simulink model "exampleModel_bus_axi_w_4ptavg"  (R2017b)
settings: Solver=VariableStepAuto  StartTime=0.0  StopTime=10e-5  RelTol=1e-3
PreLoadFcn:
  | setup
values from neighbouring files (symbols this model uses):
  axiClk = 156.25e6    (= 156250000)    [setup.m]    (also in setup_exampleModel_bus_axi_simulink.m; setup_exampleModel_bus_axi_simulink_lcls2.m; setup_lcls2_pcav.m; sysgen_signal.m)
  cav1p1_addr = 204    [setup_exampleModel_bus_axi_simulink.m]    (also in setup_exampleModel_bus_axi_simulink_lcls2.m; setup_lcls2_pcav.m; sysgen_signal.m)
  cav1p2_addr = cav1p1_addr * 2    (= 408)    [setup_exampleModel_bus_axi_simulink.m]    (also in setup_exampleModel_bus_axi_simulink_lcls2.m; setup_lcls2_pcav.m; sysgen_signal.m)
  cav2p1_addr = cav1p1_addr * 3    (= 612)    [setup_exampleModel_bus_axi_simulink.m]    (also in setup_exampleModel_bus_axi_simulink_lcls2.m; setup_lcls2_pcav.m; sysgen_signal.m)
  cav2p2_addr = cav1p1_addr * 4    (= 816)    [setup_exampleModel_bus_axi_simulink.m]    (also in setup_exampleModel_bus_axi_simulink_lcls2.m; setup_lcls2_pcav.m; sysgen_signal.m)
  Fadc = Fs/interleavedChannels    (= 29750000)    [setup.m]    (also in setup_exampleModel_bus_axi_simulink.m = 357000000; setup_exampleModel_bus_axi_simulink_lcls2.m = 351000000; setup_lcls2_pcav.m = 357000000; sysgen_signal.m = 357000000)
  fir_lpf = fir1(15, w_lpf)    [setup_exampleModel_bus_axi_simulink.m]    (also in setup_exampleModel_bus_axi_simulink_lcls2.m; setup_lcls2_pcav.m)
  Fproc = 204e6    (= 204000000)    [setup_exampleModel_bus_axi_simulink.m]    (also in setup_exampleModel_bus_axi_simulink_lcls2.m = 200571400; setup_lcls2_pcav.m; sysgen_signal.m)
  Fsig = Fproc/12    (= 17000000)    [setup_exampleModel_bus_axi_simulink.m]    (also in setup_exampleModel_bus_axi_simulink_lcls2.m = 16714283.3333; setup_lcls2_pcav.m)
  Tadc = 1/fadc    (= 2.80112044818e-09)    [cavity_signal.m]    (also in setup_exampleModel_bus_axi_simulink.m; setup_exampleModel_bus_axi_simulink_lcls2.m = 2.849002849e-09; setup_lcls2_pcav.m; setup_pcav_simulink.m)
undefined symbols (not defined in the file or in its folder): AXI4, Lite
libraries: xbsIndex_r4 x2870, llrf_lib x10, simulink x3
(part 5 of 15)

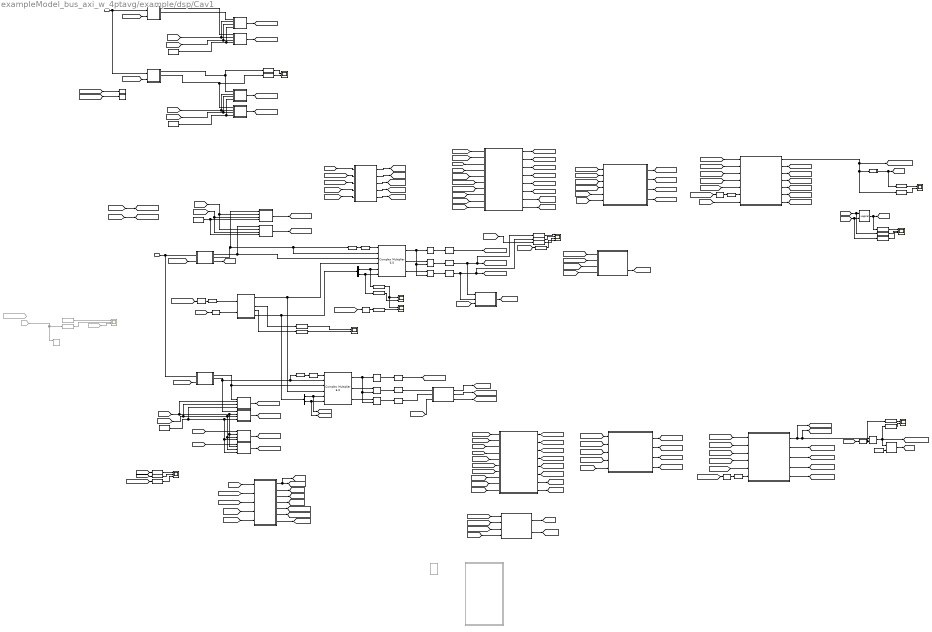
== system exampleModel_bus_axi_w_4ptavg/example/dsp/Cav1 ==
  PA_stream : Inport
  IQ_stream : Inport  Port=2
  AddSub : xbsIndex_r4/AddSub  Commented=on  mode=Addition  use_carryin=off  use_carryout=off  en=off  latency=1  precision=User Defined  arith_type=Unsigned  n_bits=32  bin_pt=32  quantization=Truncate  overflow=Saturate  use_behavioral_HDL=off  hw_selection=Fabric  pipelined=off  dbl_ovrd=off  block_type=addsub
  Bus Selector : BusSelector  OutputSignals=NCO_sin,NCO_cos
  Bus Selector1 : BusSelector  OutputSignals=NCO_sin,NCO_cos
  Clock Enable Probe : xbsIndex_r4/Clock Enable Probe  inherit_constraints=on  block_type=ceprobe
      settings: infoedit="Clock enable extractor.  Produces a Boolean output that mirrors the hardware clock enable associated with the input sample rate.<br><br>Hardware notes: in hardware this block costs nothing."
  Clock Enable Probe1 : xbsIndex_r4/Clock Enable Probe  inherit_constraints=on  block_type=ceprobe
      settings: infoedit="Clock enable extractor.  Produces a Boolean output that mirrors the hardware clock enable associated with the input sample rate.<br><br>Hardware notes: in hardware this block costs nothing."
  "Complex Multiplier 6.0 " : xbsIndex_r4/Complex Multiplier 6.0   hasatlast=off  hasatuser=off  atuserwidth=1  hasbtlast=off  hasbtuser=off  btuserwidth=1  multtype=Use_Mults  optimizegoal=Resources  flowcontrol=NonBlocking  outputwidth=33  roundmode=Truncate  hasctrltlast=off  hasctrltuser=off  ctrltuserwidth=1  outtlastbehv=Null  latencyconfig=Automatic  minimumlatency=15  aclken=off  aresetn=off  trim_axipin_name=on  simulation_type=hybrid_sim  simulation_model=sysgen:cmpy_v6_0  data_path_portlist={ 's_axis_a_tdata_real', 's_axis_a_tdata_imag', 's_axis_b_tdata_real', 's_axis_b_tdata_imag', 's_axis_ctrl_tdata_rounding_bit', 'm_axis_dout_tdata_real', 'm_axis_dout_tdata_imag' }  aportwidth=63  bportwidth=63  ip_name=Complex Multiplier  ip_version=6.0  dsptool_ready=true  ipcore_usecache=true  ipcore_useipmodelcache=true  ipcore_verbose=false  ipcore_latency_parameter='minimumlatency'  wrapper_available=true  port_translation_map={ 'aclken' => 'en', 'aresetn' => 'rst'}  block_type=cmpy_v6_0
  Complex Multiplier 6.0 1 : xbsIndex_r4/Complex Multiplier 6.0   hasatlast=off  hasatuser=off  atuserwidth=1  hasbtlast=off  hasbtuser=off  btuserwidth=1  multtype=Use_Mults  optimizegoal=Resources  flowcontrol=NonBlocking  outputwidth=21  roundmode=Truncate  hasctrltlast=off  hasctrltuser=off  ctrltuserwidth=1  outtlastbehv=Null  latencyconfig=Automatic  minimumlatency=37  aclken=off  aresetn=off  trim_axipin_name=on  simulation_type=hybrid_sim  simulation_model=sysgen:cmpy_v6_0  data_path_portlist={ 's_axis_a_tdata_real', 's_axis_a_tdata_imag', 's_axis_b_tdata_real', 's_axis_b_tdata_imag', 's_axis_ctrl_tdata_rounding_bit', 'm_axis_dout_tdata_real', 'm_axis_dout_tdata_imag' }  aportwidth=63  bportwidth=63  ip_name=Complex Multiplier  ip_version=6.0  dsptool_ready=true  ipcore_usecache=true  ipcore_useipmodelcache=true  ipcore_verbose=false  ipcore_latency_parameter='minimumlatency'  wrapper_available=true  port_translation_map={ 'aclken' => 'en', 'aresetn' => 'rst'}  block_type=cmpy_v6_0
  Constant : xbsIndex_r4/Constant  const=0  gui_display_data_type=Fixed-point  arith_type=Signed (2's comp)  n_bits=1  bin_pt=0  preci_type=Single  exp_width=8  frac_width=24  explicit_period=off  period=1  equ=P=C  opselect=C  inp2=PCIN>>17  opr=+  inp1=P  carry=CIN  dbl_ovrd=off  block_type=constant
  Constant{1..4} (4 alike) : xbsIndex_r4/Constant  const=29  gui_display_data_type=Fixed-point  arith_type=Unsigned  n_bits=16  bin_pt=0  preci_type=Single  exp_width=8  frac_width=24  explicit_period=off  period=1  equ=P=C  opselect=C  inp2=PCIN>>17  opr=+  inp1=P  carry=CIN  dbl_ovrd=off  block_type=constant
  Convert{,1,5..6} (4 alike) : xbsIndex_r4/Convert  gui_display_data_type=Fixed-point  arith_type="Signed  (2's comp)"  n_bits=18  bin_pt=16  float_type=Single  exp_bits=8  fraction_bits=24  quantization=Truncate  overflow=Wrap  en=off  latency=1  pipeline=off  dbl_ovrd=off  block_type=convert
  Convert10 : xbsIndex_r4/Convert  gui_display_data_type=Boolean  arith_type=Boolean  n_bits=16  bin_pt=14  float_type=Single  exp_bits=8  fraction_bits=24  quantization=Truncate  overflow=Wrap  en=off  latency=1  pipeline=off  dbl_ovrd=off  block_type=convert
  Convert2 : xbsIndex_r4/Convert  gui_display_data_type=Boolean  arith_type=Boolean  n_bits=18  bin_pt=16  float_type=Single  exp_bits=8  fraction_bits=24  quantization=Truncate  overflow=Wrap  en=off  latency=1  pipeline=off  dbl_ovrd=off  block_type=convert
  Convert9 : xbsIndex_r4/Convert  gui_display_data_type=Boolean  arith_type=Boolean  n_bits=18  bin_pt=16  float_type=Single  exp_bits=8  fraction_bits=24  quantization=Truncate  overflow=Wrap  en=off  latency=1  pipeline=off  dbl_ovrd=off  block_type=convert
  DDC NCO1 : Subsystem
  Down Sample{1..3,6..7} (5 alike) : xbsIndex_r4/Down Sample  sample_ratio=12  sample_phase="Last Value of Frame  (most efficient)"  en=off  rst=off  latency=1  dbl_ovrd=off  block_type=dsamp
  From89 : From  Commented=on  GotoTag=cav1_p2_dc_freq  TagVisibility=global
  From90 : From  Commented=on  GotoTag=sim_f_err  TagVisibility=global
  From91 : From  Commented=on  GotoTag=testa  TagVisibility=global
  Gateway Out{1..6,8..10,25,39..40} (12 alike) : xbsIndex_r4/Gateway Out  inherit_from_input=off  hdl_port=on  rows=1  columns=1  UseAsDAC=off  DACChannel='1'  interface=None  automatic_assignment=on  address_offset=hex2dec('00')  intf_name=''  intf_description=''  timing_constraint=None  locs_specified=off  LOCs={}  io_standard={}  block_type=gatewayout
  Gateway Out{26..28,30..33} (7 alike) : xbsIndex_r4/Gateway Out  inherit_from_input=off  hdl_port=off  rows=1  columns=1  UseAsDAC=off  DACChannel='1'  interface=None  automatic_assignment=on  address_offset=hex2dec('00')  intf_name=''  intf_description=''  timing_constraint=None  locs_specified=off  LOCs={}  io_standard={}  block_type=gatewayout
  Gateway Out36 : xbsIndex_r4/Gateway Out  Commented=on  inherit_from_input=off  hdl_port=on  rows=1  columns=1  UseAsDAC=off  DACChannel='1'  interface=None  automatic_assignment=on  address_offset=hex2dec('00')  intf_name=''  intf_description=''  timing_constraint=None  locs_specified=off  LOCs={}  io_standard={}  block_type=gatewayout
  Gateway Out37 : xbsIndex_r4/Gateway Out  Commented=on  inherit_from_input=off  hdl_port=on  rows=1  columns=1  UseAsDAC=off  DACChannel='1'  interface=None  automatic_assignment=on  address_offset=hex2dec('00')  intf_name=''  intf_description=''  timing_constraint=None  locs_specified=off  LOCs={}  io_standard={}  block_type=gatewayout
  IQ_integration : Subsystem
  IQ_integration1 : Subsystem
  Logical : xbsIndex_r4/Logical  logical_function=AND  inputs=2  en=off  latency=1  precision=Full  arith_type=Unsigned  n_bits=16  bin_pt=0  align_bp=on  dbl_ovrd=off  block_type=logical
  Masking_n_delay : Subsystem
  NCO_cos : xbsIndex_r4/Gateway Out  inherit_from_input=off  hdl_port=off  rows=1  columns=1  UseAsDAC=off  DACChannel='1'  interface=None  automatic_assignment=on  address_offset=hex2dec('00')  intf_name=''  intf_description=''  timing_constraint=None  locs_specified=off  LOCs={}  io_standard={}  block_type=gatewayout
  NCO_sin : xbsIndex_r4/Gateway Out  inherit_from_input=off  hdl_port=off  rows=1  columns=1  UseAsDAC=off  DACChannel='1'  interface=None  automatic_assignment=on  address_offset=hex2dec('00')  intf_name=''  intf_description=''  timing_constraint=None  locs_specified=off  LOCs={}  io_standard={}  block_type=gatewayout
  PA_conversion2 : Subsystem
  PA_select : Subsystem
  PA_select1 : Subsystem
  Register : xbsIndex_r4/Register  init=0  rst=on  en=off  dbl_ovrd=off  block_type=register
  Register{1..2,32..33} (4 alike) : xbsIndex_r4/Register  init=0  rst=off  en=on  dbl_ovrd=off  block_type=register
  Register{3..10,31} (9 alike) : xbsIndex_r4/Register  init=0  rst=off  en=off  dbl_ovrd=off  block_type=register
  Relational : xbsIndex_r4/Relational  mode=a!=b  op_type=Bool  en=off  latency=1  dbl_ovrd=off  block_type=relational
  Scope1 : Scope  NumInputPorts=4
  Scope{2..3,11..14} (6 alike) : Scope  NumInputPorts=2
  Scope15 : Scope  NumInputPorts=3
  Scope17 : Scope  Commented=on  NumInputPorts=3
  Scope18 : Scope  NumInputPorts=3
  Subsystem : Subsystem  Commented=on
  Subsystem1 : Subsystem
  Subsystem10 : Subsystem
  Subsystem11 : Subsystem
  Subsystem12 : Subsystem
  Subsystem13 : Subsystem
  Subsystem2 : Subsystem
  Subsystem3 : Subsystem
  Subsystem4 : Subsystem
  Subsystem5 : Subsystem
  Subsystem6 : Subsystem
  Subsystem7 : Subsystem
  Subsystem8 : Subsystem
  Subsystem9 : Subsystem
  c1p1_Masking_window : Subsystem
  c1p1_PA_conversion : Subsystem
  c1p1_freq_err_module : Subsystem
  "c1p1_window_wf1 " : Subsystem
  c1p2_freq_err_module : Subsystem
  c1p2_window_wf : Subsystem
  c1p2_window_wf1 : Subsystem  Commented=on
  c1p2_windowing_func1 : Subsystem
  c1p2_windowing_func2 : Subsystem
  tag scope: Cav1_NCO_fb=global, c1_p1_delay_amt=global, c1_p1_delay_latch=global, c1_p2_delay_amt=global, c1_p2_delay_latch=global, c1_ready=global, c1_stream_valid=global, c1p1_delay_match=global, c1p1_freq_err=global, c1p1_integral_logic=global, c1p1_pt_cntr=global, c1p1_pt_window=global, c1p1_ready=global, c1p1_window_func=global, c1p2_delay_match=global, c1p2_freq_err=global, c1p2_integral_logic=global, c1p2_pt_cntr=global, c1p2_pt_window=global, c1p2_ready=global, c1p2_window_func=global, cav1_NCO_cos=global, cav1_NCO_sin=global, cav1_p1_amp_out=global, cav1_p1_comparison_i=global, cav1_p1_comparison_phase=global, cav1_p1_comparison_q=global, cav1_p1_dc_freq=global, cav1_p1_dc_img=global, cav1_p1_dc_real=global, cav1_p1_dc_tvalid=global, cav1_p1_delayed_dc_img=global, cav1_p1_delayed_dc_real=global, cav1_p1_if_amp=global, cav1_p1_if_i=global, cav1_p1_if_phase=global, cav1_p1_if_q=global, cav1_p1_integrated_i=global, cav1_p1_integrated_q=global, cav1_p1_integrated_ref_i=global, cav1_p1_integrated_ref_q=global, cav1_p1_phase_out=global, cav1_p1_ref_amp_out=global, cav1_p1_ref_phase_out=global, cav1_p1_windowed_img=global, cav1_p1_windowed_real=global, cav1_p1_windowed_ref_i=global, cav1_p1_windowed_ref_q=global, cav1_p2_amp_out=global, cav1_p2_comparison_i=global, cav1_p2_comparison_phase=global, cav1_p2_comparison_q=global, cav1_p2_dc_freq=global, cav1_p2_dc_img=global, cav1_p2_dc_real=global, cav1_p2_dc_tvalid=global, cav1_p2_delayed_dc_img=global, cav1_p2_delayed_dc_real=global, cav1_p2_if_amp=global, cav1_p2_if_i=global, cav1_p2_if_phase=global, cav1_p2_if_q=global, cav1_p2_integrated_i=global, cav1_p2_integrated_q=global, cav1_p2_integrated_ref_i=global, cav1_p2_integrated_ref_q=global, cav1_p2_phase_out=global, cav1_p2_ref_amp_out=global, cav1_p2_ref_phase_out=global, cav1_p2_windowed_img=global, cav1_p2_windowed_real=global, cav1_p2_windowed_ref_i=global, cav1_p2_windowed_ref_q=global, cav1_sync=global, dsp_cav1_reset=global, flo_c1p1_window=global, flo_c1p2_window=global, ref_i_reg=global, ref_q_reg=global, reset=global
  wires:
  PA_select/1(Amp) -> Subsystem13/1(d)
  "Complex Multiplier 6.0 "/2 -> Register1/1
  Bus Selector/2 -> NCO_cos/1, "Complex Multiplier 6.0 "/6  "<NCO_cos>"
  "Complex Multiplier 6.0 "/3 -> Register2/1
  [cav1_nco_phase_adj] -> Register8/1
  [cav1_sync] -> Register7/1
  Bus Selector/1 -> NCO_sin/1, "Complex Multiplier 6.0 "/5  "<NCO_sin>"
  DDC NCO1/5(NCO_out) -> Bus Selector1/1, Bus Selector/1
  PA_select/2(Phase) -> Subsystem12/1(d)  "phase"
  Subsystem3/2(ddcQ) -> Subsystem6/1(d), "Complex Multiplier 6.0 "/2, Clock Enable Probe/1  "ddcQ"
  Subsystem3/1(ddcI) -> Subsystem7/1(d), "Complex Multiplier 6.0 "/3  "ddcI"
  NCO_cos/1 -> Scope11/2
  NCO_sin/1 -> Scope12/1, Scope11/1
  Clock Enable Probe/1 -> Down Sample2/1
  IQ_stream/1 -> Subsystem1/1(IQ_stream_in), Subsystem3/1(IQ_stream_in)
  [cav1_p1_chan_sel] -> PA_select/2(PA_chan_sel)
  [cav1_p1_chan_sel] -> Subsystem3/2(IQ_chan_sel)
  [cav1_nco_phase_adj] -> Register9/1
  [cav1_p2_chan_sel] -> PA_select1/2(PA_chan_sel)
  PA_select1/2(Phase) -> Gateway Out9/1, Subsystem11/1(d)  "phase"
  PA_select1/1(Amp) -> Gateway Out8/1, Subsystem10/1(d)
  PA_stream/1 -> PA_select1/1(PA_bus), PA_select/1(PA_bus)
  [cav1_p2_chan_sel] -> Subsystem1/2(IQ_chan_sel)
  Complex Multiplier 6.0 1/2 -> Register32/1
  Register31/1 -> Convert2/1
  Complex Multiplier 6.0 1/1 -> Register33/2, Register32/2, Register31/1
  Bus Selector1/2 -> [cav1_NCO_cos], Complex Multiplier 6.0 1/6  "<NCO_cos>"
  Bus Selector1/1 -> [cav1_NCO_sin], Complex Multiplier 6.0 1/5  "<NCO_sin>"
  Complex Multiplier 6.0 1/3 -> Register33/1
  [cav1_p1_window_start] -> Register3/1
  [cav1_p1_window_stop] -> Register4/1
  [c1p1_freq_err] -> [cav1_p1_dc_freq]
  [c1p2_freq_err] -> [cav1_p2_dc_freq]
  Convert/1 -> c1p2_windowing_func2/1(imag)
  Convert1/1 -> c1p2_windowing_func2/2(real)
  Convert2/1 -> [cav1_p2_dc_tvalid]
  Gateway Out4/1 -> Scope12/2
  Register8/1 -> Down Sample6/1
  Register9/1 -> Gateway Out4/1
  Gateway Out40/1 -> Scope18/2
  Gateway Out39/1 -> Scope18/1
  [rf_ref_amp] -> Gateway Out39/1
  [rf_ref_phase] -> Gateway Out40/1
  Register33/1 -> Convert1/1
  [c1p2_pt_window] -> IQ_integration/5(window_profile)
  [cav1_p2_windowed_ref_q] -> IQ_integration/4(ref_windowed_q)
  [cav1_p2_windowed_ref_i] -> IQ_integration/3(ref_windowed_i)
  [cav1_p2_windowed_real] -> IQ_integration/2(cav_windowed_real)
  [cav1_p2_windowed_img] -> IQ_integration/1(cav_windowed_imag)
  [cav1_sync] -> Masking_n_delay/1(phi_reset_trig)
  [cav1_p2_window_start] -> Masking_n_delay/2(start_pt)
  [cav1_p2_window_stop] -> Masking_n_delay/3(stop_pt)
  Masking_n_delay/1(trig_reset) -> [reset], [dsp_cav1_reset]
  Masking_n_delay/2(counter) -> [c1p2_pt_cntr]
  Masking_n_delay/3(eval_window) -> [c1p2_pt_window]
  Masking_n_delay/4(integral_trig) -> [c1p2_integral_logic]
  IQ_integration/4(ref_int_q) -> [cav1_p2_integrated_ref_q]
  IQ_integration/3(ref_int_i) -> [cav1_p2_integrated_ref_i]
  IQ_integration/2(cav_int_i) -> [cav1_p2_integrated_i]
  IQ_integration/1(cav_int_q) -> [cav1_p2_integrated_q]
  DDC NCO1/3(Sine) -> Gateway Out3/1
  DDC NCO1/4(Cosine) -> Gateway Out5/1
  Gateway Out3/1 -> Scope2/1
  Gateway Out5/1 -> Scope2/2
  Down Sample2/1 -> "Complex Multiplier 6.0 "/1
  Clock Enable Probe1/1 -> Down Sample1/1
  Down Sample1/1 -> Complex Multiplier 6.0 1/1
  Register7/1 -> DDC NCO1/2(Phase_reset)
  Convert5/1 -> c1p2_windowing_func1/1(imag), Gateway Out1/1, [cav1_p1_dc_img]
  Convert6/1 -> c1p2_windowing_func1/2(real), Gateway Out10/1, [cav1_p1_dc_real]
  [c1p1_pt_window] -> IQ_integration1/5(window_profile)
  IQ_integration1/2(cav_int_i) -> [cav1_p1_integrated_i]
  [cav1_p1_integrated_i] -> c1p1_PA_conversion/2(cav_int_i)
  [cav1_p1_windowed_ref_q] -> IQ_integration1/4(ref_windowed_q)
  Down Sample7/1 -> c1p1_PA_conversion/6(cal_coefficient)
  [cav1_p1_integrated_q] -> c1p1_PA_conversion/1(cav_int_q)
  IQ_integration1/3(ref_int_i) -> [cav1_p1_integrated_ref_i]
  [cav1_p1_integrated_ref_i] -> c1p1_PA_conversion/4(ref_int_i)
  Register6/1 -> Down Sample7/1
  [c1p1_integral_logic] -> c1p1_PA_conversion/5(integration_trig)
  [cav1_p1_windowed_img] -> IQ_integration1/1(cav_windowed_imag)
  [cav1_p1_cal_coef] -> Register6/1
  IQ_integration1/4(ref_int_q) -> [cav1_p1_integrated_ref_q]
  [cav1_p1_integrated_ref_q] -> c1p1_PA_conversion/3(ref_int_q)
  [cav1_p1_windowed_real] -> IQ_integration1/2(cav_windowed_real)
  [cav1_p1_windowed_ref_i] -> IQ_integration1/3(ref_windowed_i)
  IQ_integration1/1(cav_int_q) -> [cav1_p1_integrated_q]
  c1p1_Masking_window/2(eval_window) -> [c1p1_pt_window]
  [cav1_p1_window_start] -> c1p1_Masking_window/2(start_pt)
  [cav1_p1_window_stop] -> c1p1_Masking_window/3(stop_pt)
  [cav1_sync] -> c1p1_Masking_window/1(phi_reset_trig)
  c1p1_Masking_window/1(counter) -> [c1p1_pt_cntr]
  c1p1_Masking_window/3(integral_trig) -> [c1p1_integral_logic]
  Register1/1 -> Convert5/1
  Register2/1 -> Convert6/1
  "Complex Multiplier 6.0 "/1 -> Register10/1, Register2/2, Register1/2
  Register10/1 -> Convert9/1
  Convert9/1 -> [cav1_p1_dc_tvalid]
  c1p1_Masking_window/4(flo_window) -> [flo_c1p1_window]
  c1p1_PA_conversion/2(ref_phi_out) -> [cav1_p1_ref_phase_out]
  c1p1_PA_conversion/3(ref_amp_out) -> [cav1_p1_ref_amp_out]
  c1p1_PA_conversion/4(cav_phi_out) -> [cav1_p1_phase_out]
  c1p1_PA_conversion/5(cav_amp_out) -> [cav1_p1_amp_out]
  Masking_n_delay/5(flo_window) -> [flo_c1p2_window]
  [cav1_p2_dc_real] -> c1p2_window_wf/2(cav_real)
  [cav1_p2_dc_img] -> c1p2_window_wf/1(cav_img)
  [rf_ref_q] -> c1p2_window_wf/3(ref_img)
  [rf_ref_i] -> c1p2_window_wf/4(ref_real)
  [c1p2_window_func] -> c1p2_window_wf/5(window_profile)
  [cav1_p2_delayed_dc_real] -> c1p2_window_wf/7(cav_delayed_real)
  [cav1_p2_delayed_dc_img] -> c1p2_window_wf/6(cav_delayed_imag)
  [c1p2_pt_cntr] -> c1p2_window_wf/10(pt_cntr)
  [c1p2_pt_window] -> c1p2_window_wf/8(pt_window)
  [c1p2_delay_match] -> c1p2_window_wf/9(delay_match_amt)
  c1p2_window_wf/7(delay_amt) -> [c1_p2_delay_amt]
  c1p2_window_wf/1(cav_windowed_imag) -> [cav1_p2_windowed_img]
  c1p2_window_wf/2(cav_windowed_real) -> [cav1_p2_windowed_real]
  c1p2_window_wf/3(ref_windowed_imag) -> [cav1_p2_windowed_ref_q]
  c1p2_window_wf/4(ref_windowed_real) -> [cav1_p2_windowed_ref_i]
  c1p2_window_wf/5(delayed_cav_dc_img) -> [cav1_p2_delayed_dc_img]
  c1p2_window_wf/6(delayed_cav_dc_real) -> [cav1_p2_delayed_dc_real]
  [cav1_p2_integrated_ref_q] -> PA_conversion2/3(ref_int_q)
  [cav1_p2_integrated_i] -> PA_conversion2/2(cav_int_i)
  [cav1_p2_integrated_q] -> PA_conversion2/1(cav_int_q)
  [cav1_p2_integrated_ref_i] -> PA_conversion2/4(ref_int_i)
  Register5/1 -> Down Sample3/1
  [cav1_p2_cal_coef] -> Register5/1
  [c1p2_integral_logic] -> PA_conversion2/5(integration_trig)
  Down Sample3/1 -> PA_conversion2/6(cal_coefficient)
  PA_conversion2/1(phi_diff) -> [cav1_p2_comparison_q], Register/1, [cav1_p2_comparison_i]
  PA_conversion2/2(ref_phi_out) -> [cav1_p2_ref_phase_out]
  PA_conversion2/3(ref_amp_out) -> [cav1_p2_ref_amp_out]
  PA_conversion2/4(cav_phi_out) -> [cav1_p2_phase_out]
  PA_conversion2/5(cav_amp_out) -> [cav1_p2_amp_out]
  c1p2_windowing_func1/1(Window_profile) -> [c1p1_window_func]
  DDC NCO1/1(tvalid) -> "Complex Multiplier 6.0 "/4, Complex Multiplier 6.0 1/4
  Subsystem3/3(sync) -> [cav1_sync]  "sync"
  [cav1_nco_phase_reset] -> Gateway Out25/1
  Gateway Out25/1 -> Scope18/3
  [cav1_sync] -> Convert10/1
  Convert10/1 -> Gateway Out26/1, Register/2
  Gateway Out26/1 -> Scope13/1
  Gateway Out27/1 -> Scope13/2
  Register/1 -> [cav1_p2_comparison_phase], Relational/1, Gateway Out27/1
  Constant/1 -> Relational/2
  Relational/1 -> [c1p2_ready]
  Subsystem2/1(Out1) -> Gateway Out28/1, [c1p1_ready]
  c1p1_PA_conversion/1(phi_diff) -> Subsystem2/1(In1), Gateway Out30/1, [cav1_p1_comparison_phase]
  [c1p1_ready] -> Gateway Out32/1, Logical/1
  [c1p2_ready] -> Gateway Out33/1, Logical/2
  Logical/1 -> Gateway Out31/1, [c1_ready]
  Gateway Out30/1 -> Scope14/2
  Gateway Out28/1 -> Scope14/1
  Gateway Out31/1 -> Scope15/1
  Gateway Out32/1 -> Scope15/2
  Gateway Out33/1 -> Scope15/3
  Masking_n_delay/6(Stream_valid) -> [c1_stream_valid]
  Down Sample6/1 -> DDC NCO1/1(Phase_ctrl)
  From91/1 -> Gateway Out37/1, AddSub/1
  Gateway Out36/1 -> Scope17/1
  Gateway Out37/1 -> Scope17/2
  ? -> Gateway Out36/1
  From90/1 -> Scope17/3
  [c1p2_pt_window] -> c1p2_windowing_func2/3(eval_window)
  c1p2_windowing_func2/1(Window_profile) -> [c1p2_window_func]
  [cav1_p2_windowed_img] -> c1p2_freq_err_module/1(imag)
  [cav1_p2_windowed_real] -> c1p2_freq_err_module/2(real)
  [flo_c1p2_window] -> c1p2_freq_err_module/3(flo_window)
  [dsp_cav1_reset] -> c1p2_freq_err_module/4(reset)
  c1p2_freq_err_module/1(NCO_err_fb) -> [Cav1_NCO_fb]
  [c1p1_pt_window] -> c1p2_windowing_func1/3(eval_window)
  [dsp_cav1_reset] -> c1p1_freq_err_module/4(reset)
  [flo_c1p1_window] -> c1p1_freq_err_module/3(flo_window)
  [cav1_p1_windowed_img] -> c1p1_freq_err_module/1(imag)
  [cav1_p1_windowed_real] -> c1p1_freq_err_module/2(real)
  c1p1_freq_err_module/2(freq_err) -> [c1p1_freq_err]
  c1p2_freq_err_module/2(freq_err) -> [c1p2_freq_err]
  [c1_p2_delay_amt] -> Masking_n_delay/4(delay_amt)
  c1p2_window_wf/8(delay_amt_latch) -> [c1_p2_delay_latch]
  [c1_p2_delay_latch] -> Masking_n_delay/5(delay_latch)
  Masking_n_delay/7(delay_val) -> [c1p2_delay_match]
  [c1p1_delay_match] -> "c1p1_window_wf1 "/9(delay_match_amt)
  [c1p1_pt_cntr] -> "c1p1_window_wf1 "/10(pt_cntr)
  [c1p1_pt_window] -> "c1p1_window_wf1 "/8(pt_window)
  [rf_ref_i] -> "c1p1_window_wf1 "/4(ref_real)
  [cav1_p1_delayed_dc_img] -> "c1p1_window_wf1 "/6(cav_delayed_imag)
  [cav1_p1_delayed_dc_real] -> "c1p1_window_wf1 "/7(cav_delayed_real)
  [cav1_p1_dc_real] -> "c1p1_window_wf1 "/2(cav_real)
  [rf_ref_q] -> "c1p1_window_wf1 "/3(ref_img)
  [c1p1_window_func] -> "c1p1_window_wf1 "/5(window_profile)
  [cav1_p1_dc_img] -> "c1p1_window_wf1 "/1(cav_img)
  "c1p1_window_wf1 "/6(delayed_cav_dc_real) -> [cav1_p1_delayed_dc_real]
  "c1p1_window_wf1 "/7(delay_amt) -> [c1_p1_delay_amt]
  "c1p1_window_wf1 "/5(delayed_cav_dc_img) -> [cav1_p1_delayed_dc_img]
  "c1p1_window_wf1 "/2(cav_windowed_real) -> [cav1_p1_windowed_real]
  "c1p1_window_wf1 "/1(cav_windowed_imag) -> [cav1_p1_windowed_img]
  "c1p1_window_wf1 "/3(ref_windowed_imag) -> [cav1_p1_windowed_ref_q]
  "c1p1_window_wf1 "/4(ref_windowed_real) -> [cav1_p1_windowed_ref_i]
  "c1p1_window_wf1 "/8(delay_amt_latch) -> [c1_p1_delay_latch]
  [c1_p1_delay_amt] -> c1p1_Masking_window/4(delay_amt)
  [c1_p1_delay_latch] -> c1p1_Masking_window/5(delay_latch)
  c1p1_Masking_window/5(delay_val) -> [c1p1_delay_match]
  Gateway Out10/1 -> Scope1/2
  Gateway Out1/1 -> Scope1/1
  c1p1_PA_conversion/6(phi_diff_Q) -> [cav1_p1_comparison_q]
  c1p1_PA_conversion/7(phi_diff_I) -> [cav1_p1_comparison_i]
  [reset] -> IQ_integration1/6(reset)
  [reset] -> c1p1_PA_conversion/7(reset)
  Gateway Out2/1 -> Scope1/3
  [c1p1_pt_window] -> Gateway Out2/1
  [c1p2_pt_cntr] -> Gateway Out6/1
  Gateway Out6/1 -> Scope1/4
  Subsystem1/2(ddcQ) -> Subsystem4/1(d), Complex Multiplier 6.0 1/2, Clock Enable Probe1/1
  [reset] -> Subsystem5/2(reset), Subsystem9/2(reset), Subsystem8/2(reset), Subsystem4/2(reset)
  [c1p2_pt_cntr] -> Subsystem5/3(cntr), Subsystem8/3(cntr), Subsystem9/3(cntr), Subsystem4/3(cntr)
  Constant1/1 -> Subsystem5/4(threshold), Subsystem9/4(threshold), Subsystem8/4(threshold), Subsystem4/4(threshold)
  Subsystem4/1(q) -> [cav1_p2_if_q]
  Subsystem5/1(q) -> [cav1_p2_if_i]
  Subsystem6/1(q) -> [cav1_p1_if_q]
  Subsystem7/1(q) -> [cav1_p1_if_i]
  [reset] -> Subsystem7/2(reset), Subsystem6/2(reset)
  [c1p2_pt_cntr] -> Subsystem7/3(cntr), Subsystem6/3(cntr)
  Constant2/1 -> Subsystem6/4(threshold), Subsystem7/4(threshold)
  [rf_ref_i] -> Subsystem8/1(d)
  [rf_ref_q] -> Subsystem9/1(d)
  Subsystem8/1(q) -> [ref_i_reg]
  Subsystem9/1(q) -> [ref_q_reg]
  [reset] -> Subsystem10/2(reset), Subsystem11/2(reset)
  Constant3/1 -> Subsystem10/4(threshold), Subsystem11/4(threshold)
  [c1p2_pt_cntr] -> Subsystem10/3(cntr), Subsystem11/3(cntr)
  Subsystem10/1(q) -> [cav1_p2_if_amp]
  Subsystem11/1(q) -> [cav1_p2_if_phase]
  Subsystem13/1(q) -> [cav1_p1_if_amp]
  [c1p2_pt_cntr] -> Subsystem12/3(cntr), Subsystem13/3(cntr)
  [reset] -> Subsystem12/2(reset), Subsystem13/2(reset)
  Subsystem12/1(q) -> [cav1_p1_if_phase]
  Constant4/1 -> Subsystem12/4(threshold), Subsystem13/4(threshold)
  Subsystem1/1(ddcI) -> Complex Multiplier 6.0 1/3, Subsystem5/1(d)
  Register32/1 -> Convert/1
  Gateway Out8/1 -> Scope3/1
  Gateway Out9/1 -> Scope3/2
  c1p2_windowing_func2/3(filtered_I) -> [cav1_p2_dc_real]
  c1p2_windowing_func2/2(filtered_Q) -> [cav1_p2_dc_img]

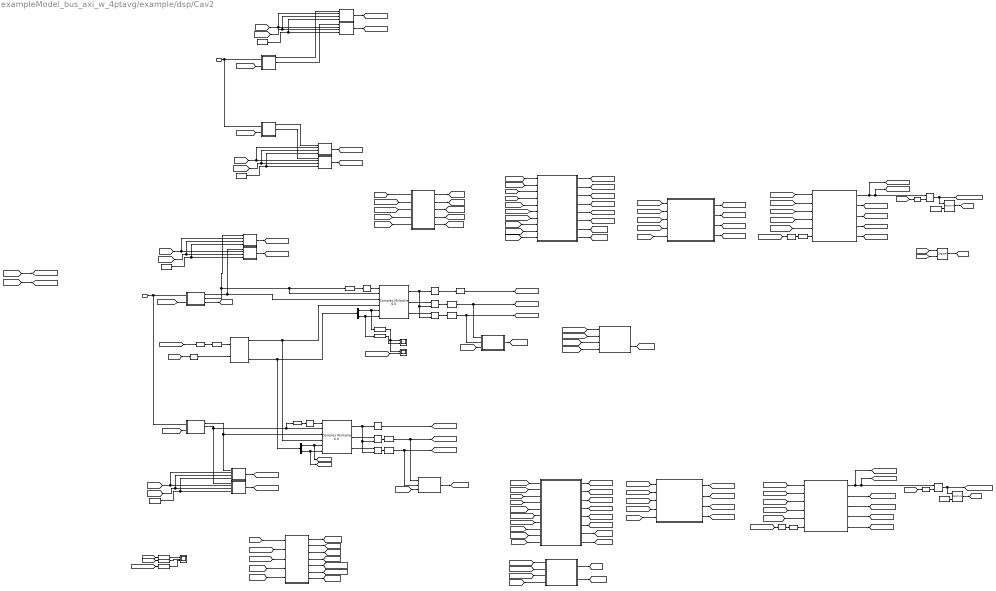
== system exampleModel_bus_axi_w_4ptavg/example/dsp/Cav2 ==
  PA_stream : Inport
  IQ_stream : Inport  Port=2
  Bus Selector : BusSelector  OutputSignals=NCO_sin,NCO_cos
  Bus Selector1 : BusSelector  OutputSignals=NCO_sin,NCO_cos
  Clock Enable Probe : xbsIndex_r4/Clock Enable Probe  inherit_constraints=on  block_type=ceprobe
      settings: infoedit="Clock enable extractor.  Produces a Boolean output that mirrors the hardware clock enable associated with the input sample rate.<br><br>Hardware notes: in hardware this block costs nothing."
  Clock Enable Probe1 : xbsIndex_r4/Clock Enable Probe  inherit_constraints=on  block_type=ceprobe
      settings: infoedit="Clock enable extractor.  Produces a Boolean output that mirrors the hardware clock enable associated with the input sample rate.<br><br>Hardware notes: in hardware this block costs nothing."
  "Complex Multiplier 6.0 " : xbsIndex_r4/Complex Multiplier 6.0   hasatlast=off  hasatuser=off  atuserwidth=1  hasbtlast=off  hasbtuser=off  btuserwidth=1  multtype=Use_Mults  optimizegoal=Resources  flowcontrol=NonBlocking  outputwidth=33  roundmode=Truncate  hasctrltlast=off  hasctrltuser=off  ctrltuserwidth=1  outtlastbehv=Null  latencyconfig=Automatic  minimumlatency=15  aclken=off  aresetn=off  trim_axipin_name=on  simulation_type=hybrid_sim  simulation_model=sysgen:cmpy_v6_0  data_path_portlist={ 's_axis_a_tdata_real', 's_axis_a_tdata_imag', 's_axis_b_tdata_real', 's_axis_b_tdata_imag', 's_axis_ctrl_tdata_rounding_bit', 'm_axis_dout_tdata_real', 'm_axis_dout_tdata_imag' }  aportwidth=63  bportwidth=63  ip_name=Complex Multiplier  ip_version=6.0  dsptool_ready=true  ipcore_usecache=true  ipcore_useipmodelcache=true  ipcore_verbose=false  ipcore_latency_parameter='minimumlatency'  wrapper_available=true  port_translation_map={ 'aclken' => 'en', 'aresetn' => 'rst'}  block_type=cmpy_v6_0
  Complex Multiplier 6.0 1 : xbsIndex_r4/Complex Multiplier 6.0   hasatlast=off  hasatuser=off  atuserwidth=1  hasbtlast=off  hasbtuser=off  btuserwidth=1  multtype=Use_Mults  optimizegoal=Resources  flowcontrol=NonBlocking  outputwidth=33  roundmode=Truncate  hasctrltlast=off  hasctrltuser=off  ctrltuserwidth=1  outtlastbehv=Null  latencyconfig=Automatic  minimumlatency=15  aclken=off  aresetn=off  trim_axipin_name=on  simulation_type=hybrid_sim  simulation_model=sysgen:cmpy_v6_0  data_path_portlist={ 's_axis_a_tdata_real', 's_axis_a_tdata_imag', 's_axis_b_tdata_real', 's_axis_b_tdata_imag', 's_axis_ctrl_tdata_rounding_bit', 'm_axis_dout_tdata_real', 'm_axis_dout_tdata_imag' }  aportwidth=63  bportwidth=63  ip_name=Complex Multiplier  ip_version=6.0  dsptool_ready=true  ipcore_usecache=true  ipcore_useipmodelcache=true  ipcore_verbose=false  ipcore_latency_parameter='minimumlatency'  wrapper_available=true  port_translation_map={ 'aclken' => 'en', 'aresetn' => 'rst'}  block_type=cmpy_v6_0
  Constant{1..2,4..5} (4 alike) : xbsIndex_r4/Constant  const=29  gui_display_data_type=Fixed-point  arith_type=Unsigned  n_bits=16  bin_pt=0  preci_type=Single  exp_width=8  frac_width=24  explicit_period=off  period=1  equ=P=C  opselect=C  inp2=PCIN>>17  opr=+  inp1=P  carry=CIN  dbl_ovrd=off  block_type=constant
  Constant3 : xbsIndex_r4/Constant  const=0  gui_display_data_type=Fixed-point  arith_type=Signed (2's comp)  n_bits=1  bin_pt=0  preci_type=Single  exp_width=8  frac_width=24  explicit_period=off  period=1  equ=P=C  opselect=C  inp2=PCIN>>17  opr=+  inp1=P  carry=CIN  dbl_ovrd=off  block_type=constant
  Constant7 : xbsIndex_r4/Constant  const=0  gui_display_data_type=Fixed-point  arith_type=Signed (2's comp)  n_bits=1  bin_pt=0  preci_type=Single  exp_width=8  frac_width=24  explicit_period=off  period=1  equ=P=C  opselect=C  inp2=PCIN>>17  opr=+  inp1=P  carry=CIN  dbl_ovrd=off  block_type=constant
  Convert{1..2,5..6} (4 alike) : xbsIndex_r4/Convert  gui_display_data_type=Fixed-point  arith_type="Signed  (2's comp)"  n_bits=18  bin_pt=16  float_type=Single  exp_bits=8  fraction_bits=24  quantization=Truncate  overflow=Wrap  en=off  latency=1  pipeline=off  dbl_ovrd=off  block_type=convert
  Convert10 : xbsIndex_r4/Convert  gui_display_data_type=Boolean  arith_type=Boolean  n_bits=16  bin_pt=14  float_type=Single  exp_bits=8  fraction_bits=24  quantization=Truncate  overflow=Wrap  en=off  latency=1  pipeline=off  dbl_ovrd=off  block_type=convert
  Convert11 : xbsIndex_r4/Convert  gui_display_data_type=Boolean  arith_type=Boolean  n_bits=16  bin_pt=14  float_type=Single  exp_bits=8  fraction_bits=24  quantization=Truncate  overflow=Wrap  en=off  latency=1  pipeline=off  dbl_ovrd=off  block_type=convert
  Convert9 : xbsIndex_r4/Convert  gui_display_data_type=Boolean  arith_type=Boolean  n_bits=18  bin_pt=16  float_type=Single  exp_bits=8  fraction_bits=24  quantization=Truncate  overflow=Wrap  en=off  latency=1  pipeline=off  dbl_ovrd=off  block_type=convert
  DDC NCO1 : Subsystem
  Down Sample{,1,3,6..7} (5 alike) : xbsIndex_r4/Down Sample  sample_ratio=12  sample_phase="Last Value of Frame  (most efficient)"  en=off  rst=off  latency=1  dbl_ovrd=off  block_type=dsamp
  Gateway Out1 : xbsIndex_r4/Gateway Out  inherit_from_input=off  hdl_port=on  rows=1  columns=1  UseAsDAC=off  DACChannel='1'  interface=None  automatic_assignment=on  address_offset=hex2dec('00')  intf_name=''  intf_description=''  timing_constraint=None  locs_specified=off  LOCs={}  io_standard={}  block_type=gatewayout
  Gateway Out39 : xbsIndex_r4/Gateway Out  inherit_from_input=off  hdl_port=on  rows=1  columns=1  UseAsDAC=off  DACChannel='1'  interface=None  automatic_assignment=on  address_offset=hex2dec('00')  intf_name=''  intf_description=''  timing_constraint=None  locs_specified=off  LOCs={}  io_standard={}  block_type=gatewayout
  Gateway Out40 : xbsIndex_r4/Gateway Out  inherit_from_input=off  hdl_port=on  rows=1  columns=1  UseAsDAC=off  DACChannel='1'  interface=None  automatic_assignment=on  address_offset=hex2dec('00')  intf_name=''  intf_description=''  timing_constraint=None  locs_specified=off  LOCs={}  io_standard={}  block_type=gatewayout
  IQ_integration : Subsystem
  IQ_integration2 : Subsystem
  Logical : xbsIndex_r4/Logical  logical_function=AND  inputs=2  en=off  latency=1  precision=Full  arith_type=Unsigned  n_bits=16  bin_pt=0  align_bp=on  dbl_ovrd=off  block_type=logical
  Masking_n_delay : Subsystem
  NCO_cos : xbsIndex_r4/Gateway Out  inherit_from_input=off  hdl_port=off  rows=1  columns=1  UseAsDAC=off  DACChannel='1'  interface=None  automatic_assignment=on  address_offset=hex2dec('00')  intf_name=''  intf_description=''  timing_constraint=None  locs_specified=off  LOCs={}  io_standard={}  block_type=gatewayout
  NCO_sin : xbsIndex_r4/Gateway Out  inherit_from_input=off  hdl_port=off  rows=1  columns=1  UseAsDAC=off  DACChannel='1'  interface=None  automatic_assignment=on  address_offset=hex2dec('00')  intf_name=''  intf_description=''  timing_constraint=None  locs_specified=off  LOCs={}  io_standard={}  block_type=gatewayout
  PA_conversion1 : Subsystem
  PA_conversion2 : Subsystem
  PA_select : Subsystem
  PA_select1 : Subsystem
  Register{,7..10,31} (6 alike) : xbsIndex_r4/Register  init=0  rst=off  en=off  dbl_ovrd=off  block_type=register
  Register{1..2,32..33} (4 alike) : xbsIndex_r4/Register  init=0  rst=off  en=on  dbl_ovrd=off  block_type=register
  Register11 : xbsIndex_r4/Register  init=0  rst=on  en=off  dbl_ovrd=off  block_type=register
  Register3 : xbsIndex_r4/Register  init=0  rst=on  en=off  dbl_ovrd=off  block_type=register
  Relational1 : xbsIndex_r4/Relational  mode=a!=b  op_type=Bool  en=off  latency=1  dbl_ovrd=off  block_type=relational
  Relational2 : xbsIndex_r4/Relational  mode=a!=b  op_type=Bool  en=off  latency=1  dbl_ovrd=off  block_type=relational
  Scope11 : Scope  NumInputPorts=2
  Scope12 : Scope  NumInputPorts=2
  Scope18 : Scope  NumInputPorts=3
  Subsystem1 : Subsystem
  Subsystem10 : Subsystem
  Subsystem11 : Subsystem
  Subsystem12 : Subsystem
  Subsystem2 : Subsystem
  Subsystem3 : Subsystem
  Subsystem4 : Subsystem
  Subsystem5 : Subsystem
  Subsystem6 : Subsystem
  Subsystem7 : Subsystem
  Subsystem8 : Subsystem
  Subsystem9 : Subsystem
  c1p2_windowing_func2 : Subsystem
  c1p2_windowing_func3 : Subsystem
  c2p1_Masking_window1 : Subsystem
  "c2p1_window_wf " : Subsystem
  c2p2_window_wf : Subsystem
  tag scope: Cav2_NCO_fb=global, c2_p1_delay_amt=global, c2_p1_delay_latch=global, c2_p2_delay_amt=global, c2_p2_delay_latch=global, c2_ready=global, c2_stream_valid=global, c2p1_delay_match=global, c2p1_freq_err=global, c2p1_integral_logic=global, c2p1_pt_cntr=global, c2p1_pt_window=global, c2p1_ready=global, c2p1_window_func=global, c2p2_delay_match=global, c2p2_freq_err=global, c2p2_integral_logic=global, c2p2_pt_cntr=global, c2p2_pt_window=global, c2p2_ready=global, c2p2_window_func=global, cav2_NCO_cos=global, cav2_NCO_sin=global, cav2_p1_amp_out=global, cav2_p1_comparison_i=global, cav2_p1_comparison_phase=global, cav2_p1_comparison_q=global, cav2_p1_dc_freq=global, cav2_p1_dc_img=global, cav2_p1_dc_real=global, cav2_p1_dc_tvalid=global, cav2_p1_delayed_dc_img=global, cav2_p1_delayed_dc_real=global, cav2_p1_if_amp=global, cav2_p1_if_i=global, cav2_p1_if_phase=global, cav2_p1_if_q=global, cav2_p1_integrated_i=global, cav2_p1_integrated_q=global, cav2_p1_integrated_ref_i=global, cav2_p1_integrated_ref_q=global, cav2_p1_phase_out=global, cav2_p1_ref_amp_out=global, cav2_p1_ref_phase_out=global, cav2_p1_windowed_img=global, cav2_p1_windowed_real=global, cav2_p1_windowed_ref_i=global, cav2_p1_windowed_ref_q=global, cav2_p2_amp_out=global, cav2_p2_comparison_i=global, cav2_p2_comparison_phase=global, cav2_p2_comparison_q=global, cav2_p2_dc_freq=global, cav2_p2_dc_img=global, cav2_p2_dc_real=global, cav2_p2_dc_tvalid=global, cav2_p2_delayed_dc_img=global, cav2_p2_delayed_dc_real=global, cav2_p2_if_amp=global, cav2_p2_if_i=global, cav2_p2_if_phase=global, cav2_p2_if_q=global, cav2_p2_integrated_i=global, cav2_p2_integrated_q=global, cav2_p2_integrated_ref_i=global, cav2_p2_integrated_ref_q=global, cav2_p2_phase_out=global, cav2_p2_ref_amp_out=global, cav2_p2_ref_phase_out=global, cav2_p2_windowed_img=global, cav2_p2_windowed_real=global, cav2_p2_windowed_ref_i=global, cav2_p2_windowed_ref_q=global, cav2_sync=global, dsp_cav2_reset=global, flo_c2p1_window=global, flo_c2p2_window=global
  wires:
  [c2p2_freq_err] -> [cav2_p2_dc_freq]
  [c2p1_freq_err] -> [cav2_p1_dc_freq]
  Subsystem1/1(ddcI) -> Complex Multiplier 6.0 1/3, Subsystem6/1(d)
  Complex Multiplier 6.0 1/3 -> Register33/1
  Bus Selector1/1 -> [cav2_NCO_sin], Complex Multiplier 6.0 1/5  "<NCO_sin>"
  Bus Selector1/2 -> [cav2_NCO_cos], Complex Multiplier 6.0 1/6  "<NCO_cos>"
  Complex Multiplier 6.0 1/1 -> Register31/1, Register32/2, Register33/2
  Register31/1 -> [cav2_p2_dc_tvalid]
  Clock Enable Probe1/1 -> Down Sample1/1
  Complex Multiplier 6.0 1/2 -> Register32/1
  [cav2_p2_chan_sel] -> Subsystem1/2(IQ_chan_sel)
  PA_stream/1 -> PA_select/1(PA_bus), PA_select1/1(PA_bus)
  PA_select1/1(Amp) -> Subsystem11/1(d)
  PA_select1/2(Phase) -> Subsystem12/1(d)  "phase"
  [cav2_p2_chan_sel] -> PA_select1/2(PA_chan_sel)
  [cav2_nco_phase_adj] -> Scope12/2
  [cav2_p1_chan_sel] -> Subsystem3/2(IQ_chan_sel)
  [cav2_p1_chan_sel] -> PA_select/2(PA_chan_sel)
  IQ_stream/1 -> Subsystem3/1(IQ_stream_in), Subsystem1/1(IQ_stream_in)
  Clock Enable Probe/1 -> Down Sample/1
  NCO_sin/1 -> Scope11/1, Scope12/1
  NCO_cos/1 -> Scope11/2
  Subsystem3/1(ddcI) -> "Complex Multiplier 6.0 "/3, Subsystem7/1(d)  "ddcI"
  Subsystem3/2(ddcQ) -> "Complex Multiplier 6.0 "/2, Clock Enable Probe/1, Subsystem8/1(d)  "ddcQ"
  PA_select/2(Phase) -> Subsystem9/1(d)  "phase"
  Register/1 -> Convert9/1
  DDC NCO1/5(NCO_out) -> Bus Selector/1, Bus Selector1/1
  Bus Selector/1 -> "Complex Multiplier 6.0 "/5, NCO_sin/1  "<NCO_sin>"
  "Complex Multiplier 6.0 "/1 -> Register/1, Register1/2, Register2/2
  "Complex Multiplier 6.0 "/3 -> Register2/1
  Bus Selector/2 -> "Complex Multiplier 6.0 "/6, NCO_cos/1  "<NCO_cos>"
  "Complex Multiplier 6.0 "/2 -> Register1/1
  PA_select/1(Amp) -> Subsystem10/1(d)
  [cav2_p1_windowed_ref_i] -> IQ_integration2/3(ref_windowed_i)
  PA_conversion1/3(ref_amp_out) -> [cav2_p1_ref_amp_out]
  [cav2_p1_integrated_ref_q] -> PA_conversion1/3(ref_int_q)
  [cav2_p1_cal_coef] -> Register7/1
  PA_conversion1/4(cav_phi_out) -> [cav2_p1_phase_out]
  [c2p1_pt_window] -> IQ_integration2/5(window_profile)
  Register7/1 -> Down Sample7/1
  PA_conversion1/1(phi_diff) -> [cav2_p1_comparison_q], Register11/1, [cav2_p1_comparison_i]
  Down Sample7/1 -> PA_conversion1/6(cal_coefficient)
  IQ_integration2/4(ref_int_q) -> [cav2_p1_integrated_ref_q]
  [cav2_p1_integrated_i] -> PA_conversion1/2(cav_int_i)
  IQ_integration2/1(cav_int_q) -> [cav2_p1_integrated_q]
  IQ_integration2/3(ref_int_i) -> [cav2_p1_integrated_ref_i]
  PA_conversion1/5(cav_amp_out) -> [cav2_p1_amp_out]
  [cav2_p1_integrated_q] -> PA_conversion1/1(cav_int_q)
  [cav2_p1_windowed_ref_q] -> IQ_integration2/4(ref_windowed_q)
  [c2p1_integral_logic] -> PA_conversion1/5(integration_trig)
  [cav2_p1_windowed_real] -> IQ_integration2/2(cav_windowed_real)
  [cav2_p1_integrated_ref_i] -> PA_conversion1/4(ref_int_i)
  IQ_integration2/2(cav_int_i) -> [cav2_p1_integrated_i]
  [cav2_p1_windowed_img] -> IQ_integration2/1(cav_windowed_imag)
  PA_conversion1/2(ref_phi_out) -> [cav2_p1_ref_phase_out]
  Register9/1 -> Down Sample6/1
  Down Sample6/1 -> DDC NCO1/1(Phase_ctrl)
  [cav2_nco_phase_adj] -> Register9/1
  [cav2_sync] -> Register8/1
  Register1/1 -> Convert5/1
  Register2/1 -> Convert1/1
  [rf_ref_phase] -> Gateway Out40/1
  Gateway Out39/1 -> Scope18/1
  [rf_ref_amp] -> Gateway Out39/1
  Gateway Out40/1 -> Scope18/2
  IQ_integration/2(cav_int_i) -> [cav2_p2_integrated_i]
  IQ_integration/3(ref_int_i) -> [cav2_p2_integrated_ref_i]
  [cav2_p2_windowed_ref_i] -> IQ_integration/3(ref_windowed_i)
  [cav2_p2_integrated_ref_i] -> PA_conversion2/4(ref_int_i)
  Register32/1 -> Convert2/1
  Register10/1 -> Down Sample3/1
  PA_conversion2/5(cav_amp_out) -> [cav2_p2_amp_out]
  [cav2_p2_windowed_img] -> IQ_integration/1(cav_windowed_imag)
  [c2p2_integral_logic] -> PA_conversion2/5(integration_trig)
  IQ_integration/1(cav_int_q) -> [cav2_p2_integrated_q]
  PA_conversion2/2(ref_phi_out) -> [cav2_p2_ref_phase_out]
  [cav2_p2_windowed_ref_q] -> IQ_integration/4(ref_windowed_q)
  PA_conversion2/3(ref_amp_out) -> [cav2_p2_ref_amp_out]
  PA_conversion2/4(cav_phi_out) -> [cav2_p2_phase_out]
  Register33/1 -> Convert6/1
  [cav2_p2_windowed_real] -> IQ_integration/2(cav_windowed_real)
  [c2p2_pt_window] -> IQ_integration/5(window_profile)
  PA_conversion2/1(phi_diff) -> [cav2_p2_comparison_i], Register3/1, [cav2_p2_comparison_q]
  [cav2_p2_integrated_i] -> PA_conversion2/2(cav_int_i)
  [cav2_p2_cal_coef] -> Register10/1
  IQ_integration/4(ref_int_q) -> [cav2_p2_integrated_ref_q]
  [cav2_p2_integrated_q] -> PA_conversion2/1(cav_int_q)
  [cav2_p2_integrated_ref_q] -> PA_conversion2/3(ref_int_q)
  Down Sample3/1 -> PA_conversion2/6(cal_coefficient)
  Convert9/1 -> [cav2_p1_dc_tvalid]
  Convert2/1 -> c1p2_windowing_func2/1(imag), [cav2_p2_dc_img]
  Convert6/1 -> c1p2_windowing_func2/2(real), [cav2_p2_dc_real]
  Down Sample/1 -> "Complex Multiplier 6.0 "/1
  Down Sample1/1 -> Complex Multiplier 6.0 1/1
  DDC NCO1/1(tvalid) -> "Complex Multiplier 6.0 "/4, Complex Multiplier 6.0 1/4
  Subsystem3/3(sync) -> [cav2_sync]  "sync"
  [cav2_nco_phase_reset] -> Gateway Out1/1
  Gateway Out1/1 -> Scope18/3
  [cav2_sync] -> Convert11/1
  Convert11/1 -> Register11/2
  Register11/1 -> Relational1/1, [cav2_p1_comparison_phase]
  Constant7/1 -> Relational1/2
  [c2p2_ready] -> Logical/2
  [c2p1_ready] -> Logical/1
  Logical/1 -> [c2_ready]
  Relational1/1 -> [c2p1_ready]
  Convert10/1 -> Register3/2
  Constant3/1 -> Relational2/2
  Relational2/1 -> [c2p2_ready]
  [cav2_sync] -> Convert10/1
  Register3/1 -> Relational2/1, [cav2_p2_comparison_phase]
  [cav2_sync] -> Masking_n_delay/1(phi_reset_trig)
  [cav2_p2_window_start] -> Masking_n_delay/2(start_pt)
  [cav2_p2_window_stop] -> Masking_n_delay/3(stop_pt)
  Masking_n_delay/1(trig_reset) -> [dsp_cav2_reset]
  Masking_n_delay/2(counter) -> [c2p2_pt_cntr]
  Masking_n_delay/3(eval_window) -> [c2p2_pt_window]
  Masking_n_delay/4(integral_trig) -> [c2p2_integral_logic]
  Masking_n_delay/5(flo_window) -> [flo_c2p2_window]
  Masking_n_delay/6(Stream_valid) -> [c2_stream_valid]
  [c2_p2_delay_amt] -> Masking_n_delay/4(delay_amt)
  Masking_n_delay/7(delay_val) -> [c2p2_delay_match]
  [c2p2_pt_window] -> c1p2_windowing_func2/3(eval_window)
  c1p2_windowing_func2/1(Window_profile) -> [c2p2_window_func]
  [cav2_p2_windowed_img] -> Subsystem2/1(imag)
  [cav2_p2_windowed_real] -> Subsystem2/2(real)
  [dsp_cav2_reset] -> Subsystem2/4(reset)
  Subsystem2/1(NCO_err_fb) -> [Cav2_NCO_fb]
  Subsystem2/2(freq_err) -> [c2p2_freq_err]
  [flo_c2p2_window] -> Subsystem2/3(flo_window)
  c2p2_window_wf/8(delay_amt_latch) -> [c2_p2_delay_latch]
  c2p2_window_wf/7(delay_amt) -> [c2_p2_delay_amt]
  c2p2_window_wf/6(delayed_cav_dc_real) -> [cav2_p2_delayed_dc_real]
  c2p2_window_wf/5(delayed_cav_dc_img) -> [cav2_p2_delayed_dc_img]
  c2p2_window_wf/4(ref_windowed_real) -> [cav2_p2_windowed_ref_i]
  c2p2_window_wf/3(ref_windowed_imag) -> [cav2_p2_windowed_ref_q]
  c2p2_window_wf/2(cav_windowed_real) -> [cav2_p2_windowed_real]
  c2p2_window_wf/1(cav_windowed_imag) -> [cav2_p2_windowed_img]
  [cav2_p2_delayed_dc_img] -> c2p2_window_wf/6(cav_delayed_imag)
  [cav2_p2_delayed_dc_real] -> c2p2_window_wf/7(cav_delayed_real)
  [c2p2_pt_cntr] -> c2p2_window_wf/10(pt_cntr)
  [c2p2_delay_match] -> c2p2_window_wf/9(delay_match_amt)
  [c2p2_pt_window] -> c2p2_window_wf/8(pt_window)
  [c2p2_window_func] -> c2p2_window_wf/5(window_profile)
  [rf_ref_i] -> c2p2_window_wf/4(ref_real)
  [rf_ref_q] -> c2p2_window_wf/3(ref_img)
  [cav2_p2_dc_real] -> c2p2_window_wf/2(cav_real)
  [cav2_p2_dc_img] -> c2p2_window_wf/1(cav_img)
  [c2_p2_delay_latch] -> Masking_n_delay/5(delay_latch)
  [cav2_sync] -> c2p1_Masking_window1/1(phi_reset_trig)
  [cav2_p1_window_start] -> c2p1_Masking_window1/2(start_pt)
  [cav2_p1_window_stop] -> c2p1_Masking_window1/3(stop_pt)
  c2p1_Masking_window1/5(delay_val) -> [c2p1_delay_match]
  [c2_p1_delay_amt] -> c2p1_Masking_window1/4(delay_amt)
  c2p1_Masking_window1/1(counter) -> [c2p1_pt_cntr]
  c2p1_Masking_window1/3(integral_trig) -> [c2p1_integral_logic]
  c2p1_Masking_window1/4(flo_window) -> [flo_c2p1_window]
  c2p1_Masking_window1/2(eval_window) -> [c2p1_pt_window]
  [cav2_p1_windowed_img] -> Subsystem4/1(imag)
  [cav2_p1_windowed_real] -> Subsystem4/2(real)
  Subsystem4/2(freq_err) -> [c2p1_freq_err]
  [flo_c2p1_window] -> Subsystem4/3(flo_window)
  Convert5/1 -> c1p2_windowing_func3/1(imag), [cav2_p1_dc_img]
  Convert1/1 -> c1p2_windowing_func3/2(real), [cav2_p1_dc_real]
  c1p2_windowing_func3/1(Window_profile) -> [c2p1_window_func]
  [c2p1_pt_window] -> c1p2_windowing_func3/3(eval_window)
  [dsp_cav2_reset] -> Subsystem4/4(reset)
  "c2p1_window_wf "/8(delay_amt_latch) -> [c2_p1_delay_latch]
  [c2_p1_delay_latch] -> c2p1_Masking_window1/5(delay_latch)
  "c2p1_window_wf "/3(ref_windowed_imag) -> [cav2_p1_windowed_ref_q]
  "c2p1_window_wf "/4(ref_windowed_real) -> [cav2_p1_windowed_ref_i]
  "c2p1_window_wf "/5(delayed_cav_dc_img) -> [cav2_p1_delayed_dc_img]
  "c2p1_window_wf "/6(delayed_cav_dc_real) -> [cav2_p1_delayed_dc_real]
  "c2p1_window_wf "/7(delay_amt) -> [c2_p1_delay_amt]
  "c2p1_window_wf "/2(cav_windowed_real) -> [cav2_p1_windowed_real]
  "c2p1_window_wf "/1(cav_windowed_imag) -> [cav2_p1_windowed_img]
  [c2p1_pt_cntr] -> "c2p1_window_wf "/10(pt_cntr)
  [c2p1_delay_match] -> "c2p1_window_wf "/9(delay_match_amt)
  [c2p1_pt_window] -> "c2p1_window_wf "/8(pt_window)
  [cav2_p1_delayed_dc_real] -> "c2p1_window_wf "/7(cav_delayed_real)
  [cav2_p1_delayed_dc_img] -> "c2p1_window_wf "/6(cav_delayed_imag)
  [c2p1_window_func] -> "c2p1_window_wf "/5(window_profile)
  [rf_ref_i] -> "c2p1_window_wf "/4(ref_real)
  [rf_ref_q] -> "c2p1_window_wf "/3(ref_img)
  [cav2_p1_dc_real] -> "c2p1_window_wf "/2(cav_real)
  [cav2_p1_dc_img] -> "c2p1_window_wf "/1(cav_img)
  Register8/1 -> DDC NCO1/2(Phase_reset)
  [reset] -> Subsystem6/2(reset), Subsystem5/2(reset)
  Constant1/1 -> Subsystem6/4(threshold), Subsystem5/4(threshold)
  [c1p2_pt_cntr] -> Subsystem6/3(cntr), Subsystem5/3(cntr)
  Subsystem1/2(ddcQ) -> Subsystem5/1(d), Complex Multiplier 6.0 1/2, Clock Enable Probe1/1
  Subsystem5/1(q) -> [cav2_p2_if_q]
  Subsystem6/1(q) -> [cav2_p2_if_i]
  [c1p2_pt_cntr] -> Subsystem8/3(cntr), Subsystem7/3(cntr)
  [reset] -> Subsystem8/2(reset), Subsystem7/2(reset)
  Constant2/1 -> Subsystem8/4(threshold), Subsystem7/4(threshold)
  Subsystem8/1(q) -> [cav2_p1_if_q]
  Subsystem7/1(q) -> [cav2_p1_if_i]
  Constant4/1 -> Subsystem10/4(threshold), Subsystem9/4(threshold)
  [c1p2_pt_cntr] -> Subsystem10/3(cntr), Subsystem9/3(cntr)
  [reset] -> Subsystem10/2(reset), Subsystem9/2(reset)
  Subsystem10/1(q) -> [cav2_p1_if_amp]
  Subsystem9/1(q) -> [cav2_p1_if_phase]
  [reset] -> Subsystem11/2(reset), Subsystem12/2(reset)
  [c1p2_pt_cntr] -> Subsystem11/3(cntr), Subsystem12/3(cntr)
  Constant5/1 -> Subsystem11/4(threshold), Subsystem12/4(threshold)
  Subsystem11/1(q) -> [cav2_p2_if_amp]
  Subsystem12/1(q) -> [cav2_p2_if_phase]
